simulink model "ECU_Arch0"  (R2022b)
settings: Solver=FixedStepDiscrete  StartTime=0.0  StopTime=10.0  RelTol=1e-3
model workspace (MAT data in the model file):
  AlignmentIdRef = Simulink.Parameter
  AlignmentIdRef.Value = 0.3
  AlignmentIdRef.Description = 'The required IdRef ( which applaies a voltage vector) to aligne the rotor to detect the encoder or resolver offset'
  AlignmentIdRef.DataType = 'single'
  AlignmentIdRef.Min = 0.1
  AlignmentIdRef.Max = 100
  AlignmentIdRef.DocUnits = 'A'
  AlignmentIdRef.Complexity = 'real'
  AlignmentIdRef.Dimensions = [1 1]
  Alignment_ReqTime_sec = Simulink.Parameter
  Alignment_ReqTime_sec.Value = 3
  Alignment_ReqTime_sec.DataType = 'single'
  Alignment_ReqTime_sec.Min = 0
  Alignment_ReqTime_sec.Max = 20
  Alignment_ReqTime_sec.Complexity = 'real'
  Alignment_ReqTime_sec.Dimensions = [1 1]
  AliveCounterStartGD = Simulink.Signal
  AliveCounterStartGD.Description = 'Alive counter to check the length of the Init of GateDriver'
  AliveCounterStartGD.DataType = 'single'
  AliveCounterStartGD.Min = -1000000
  AliveCounterStartGD.Max = 1000000
  AliveCounterStartGD.DocUnits = '-'
  AliveCounterStartGD.Dimensions = -1
  AliveCounterStartGD.DimensionsMode = 'auto'
  AliveCounterStartGD.Complexity = 'auto'
  AliveCounterStartGD.SampleTime = -1
  AliveCounterStartGD.SamplingMode = 'auto'
  AliveCounterStartGD.InitialValue = '0'
  AngleChangeDir = Simulink.Parameter
  AngleChangeDir.Value = 1
  AngleChangeDir.Description = 'It can be used to change the direction of the postion signal, but by default = 1'
  AngleChangeDir.DataType = 'single'
  AngleChangeDir.Min = -1
  AngleChangeDir.Max = 1
  AngleChangeDir.Complexity = 'real'
  AngleChangeDir.Dimensions = [1 1]
  C_LST = 0.0001
  CtrlMode = Simulink.Parameter
  CtrlMode.Value = 1
  CtrlMode.DataType = 'single'
  CtrlMode.Min = 0
  CtrlMode.Max = 1
  CtrlMode.Complexity = 'real'
  CtrlMode.Dimensions = [1 1]
  DelayTimeAfterOL_sec = Simulink.Parameter
  DelayTimeAfterOL_sec.Value = 5
  DelayTimeAfterOL_sec.DataType = 'single'
  DelayTimeAfterOL_sec.Min = 0
  DelayTimeAfterOL_sec.Max = 100
  DelayTimeAfterOL_sec.Complexity = 'real'
  DelayTimeAfterOL_sec.Dimensions = [1 1]
  DisablePWM = Simulink.Parameter
  DisablePWM.Value = 0
  DisablePWM.Description = 'Disable the PWM during the Rotor Offset Calibration'
  DisablePWM.DataType = 'single'
  DisablePWM.Min = 0
  DisablePWM.Max = 1
  DisablePWM.Complexity = 'real'
  DisablePWM.Dimensions = [1 1]
  DisablePWM_Selector = Simulink.Parameter
  DisablePWM_Selector.Value = 0
  DisablePWM_Selector.Description = 'select either without or with Disable the PWM during the Rotor Offset Calibration'
  DisablePWM_Selector.DataType = 'uint8'
  DisablePWM_Selector.Min = 0
  DisablePWM_Selector.Max = 1
  DisablePWM_Selector.DocUnits = '-'
  DisablePWM_Selector.Complexity = 'real'
  DisablePWM_Selector.Dimensions = [1 1]
  ExecutionTimeFastLoop_FOC = Simulink.Parameter
  ExecutionTimeFastLoop_FOC.Value = 0
  ExecutionTimeFastLoop_FOC.Description = 'to measure the execution time of the subsystem'
  ExecutionTimeFastLoop_FOC.DataType = 'single'
  ExecutionTimeFastLoop_FOC.Min = 0
  ExecutionTimeFastLoop_FOC.Max = 1000000
  ExecutionTimeFastLoop_FOC.Complexity = 'real'
  ExecutionTimeFastLoop_FOC.Dimensions = [1 1]
  IDcFilterConst = Simulink.Parameter
  IDcFilterConst.Value = 0.001
  IDcFilterConst.Description = 'Time constant of the FIR IDc current filter '
  IDcFilterConst.DataType = 'single'
  IDcFilterConst.Min = 0
  IDcFilterConst.Max = 1
  IDcFilterConst.Complexity = 'real'
  IDcFilterConst.Dimensions = [1 1]
  IDcFilterSelector = Simulink.Parameter
  IDcFilterSelector.Value = 0
  IDcFilterSelector.Description = 'Switch to select one of the applied IDc current filter '
  IDcFilterSelector.DataType = 'uint16'
  IDcFilterSelector.Min = 0
  IDcFilterSelector.Max = 1
  IDcFilterSelector.Complexity = 'real'
  IDcFilterSelector.Dimensions = [1 1]
  IDcOvercurrent = Simulink.Parameter
  IDcOvercurrent.Value = 5
  IDcOvercurrent.Description = 'value of the overcurrent'
  IDcOvercurrent.DataType = 'single'
  IDcOvercurrent.Min = 0.1
  IDcOvercurrent.Max = 100
  IDcOvercurrent.DocUnits = 'A'
  IDcOvercurrent.Complexity = 'real'
  IDcOvercurrent.Dimensions = [1 1]
  IDcOvercurrentAlignment = Simulink.Parameter
  IDcOvercurrentAlignment.Value = 6
  IDcOvercurrentAlignment.Description = 'Idc overcurrent limit during rotor alignment to detect the encoder or resolver offset'
  IDcOvercurrentAlignment.DataType = 'single'
  IDcOvercurrentAlignment.Min = 0.1
  IDcOvercurrentAlignment.Max = 100
  IDcOvercurrentAlignment.DocUnits = 'A'
  IDcOvercurrentAlignment.Complexity = 'real'
  IDcOvercurrentAlignment.Dimensions = [1 1]
  IQ_REF = Simulink.Signal
  IQ_REF.Description = 'The reference iq'
  IQ_REF.DataType = 'single'
  IQ_REF.Min = -100
  IQ_REF.Max = 100
  IQ_REF.DocUnits = 'A'
  IQ_REF.Dimensions = -1
  IQ_REF.DimensionsMode = 'auto'
  IQ_REF.Complexity = 'real'
  IQ_REF.SampleTime = -1
  IQ_REF.SamplingMode = 'auto'
  IQ_REF.InitialValue = '0'
  IQ_REF_MAX = Simulink.Parameter
  IQ_REF_MAX.Value = 2.3
  IQ_REF_MAX.Description = 'Maximum allowed Iq current to limit the output of the speed controller'
  IQ_REF_MAX.DataType = 'single'
  IQ_REF_MAX.Min = -100
  IQ_REF_MAX.Max = 100
  IQ_REF_MAX.DocUnits = 'A'
  IQ_REF_MAX.Complexity = 'real'
  IQ_REF_MAX.Dimensions = [1 1]
  I_MAX = Simulink.Parameter
  I_MAX.Value = 20.625
  I_MAX.Description = 'Maximum current used for current measurement scaling calibration'
  I_MAX.DataType = 'single'
  I_MAX.Min = -100
  I_MAX.Max = 100
  I_MAX.DocUnits = 'A'
  I_MAX.Complexity = 'real'
  I_MAX.Dimensions = [1 1]
  KiId = Simulink.Parameter
  KiId.Value = 0.5
  KiId.Description = 'proportional parameter Kp of the ID-current controller'
  KiId.DataType = 'single'
  KiId.Min = 0
  KiId.Max = 1000
  KiId.Complexity = 'real'
  KiId.Dimensions = [1 1]
  KiIq = Simulink.Parameter
  KiIq.Value = 0.5
  KiIq.Description = 'proportional parameter Kp of the IQ-current controller'
  KiIq.DataType = 'single'
  KiIq.Min = 0
  KiIq.Max = 1000
  KiIq.Complexity = 'real'
  KiIq.Dimensions = [1 1]
  KiSpd = Simulink.Parameter
  KiSpd.Value = 1
  KiSpd.Description = 'propotinal factor of speed controller'
  KiSpd.DataType = 'single'
  KiSpd.Min = 0
  KiSpd.Max = 1000
  KiSpd.Complexity = 'real'
  KiSpd.Dimensions = [1 1]
  KiSpdOrg = Simulink.Parameter
  KiSpdOrg.Value = 2.2316799098e-05
  KiSpdOrg.Description = 'propotinal factor of speed controller'
  KiSpdOrg.DataType = 'single'
  KiSpdOrg.Min = 0
  KiSpdOrg.Max = 1000
  KiSpdOrg.Complexity = 'real'
  KiSpdOrg.Dimensions = [1 1]
  KpId = Simulink.Parameter
  KpId.Value = 0.3
  KpId.Description = 'proportional parameter Kp of the ID-current controller'
  KpId.DataType = 'single'
  KpId.Min = 0
  KpId.Max = 1000
  KpId.Complexity = 'real'
  KpId.Dimensions = [1 1]
  KpIq = Simulink.Parameter
  KpIq.Value = 0.3
  KpIq.Description = 'proportional parameter Kp of the IQ-current controller'
  KpIq.DataType = 'single'
  KpIq.Min = 0
  KpIq.Max = 1000
  KpIq.Complexity = 'real'
  KpIq.Dimensions = [1 1]
  KpSpd = Simulink.Parameter
  KpSpd.Value = 1.5
  KpSpd.Description = 'propotinal factor of speed controller'
  KpSpd.DataType = 'single'
  KpSpd.Min = 0
  KpSpd.Max = 1000
  KpSpd.Complexity = 'real'
  KpSpd.Dimensions = [1 1]
  KpSpdOrg = Simulink.Parameter
  KpSpdOrg.Value = 0.0142073155617
  KpSpdOrg.Description = 'propotinal factor of speed controller'
  KpSpdOrg.DataType = 'single'
  KpSpdOrg.Min = 0
  KpSpdOrg.Max = 1000
  KpSpdOrg.Complexity = 'real'
  KpSpdOrg.Dimensions = [1 1]
  Low_TQLimit_SpdCtrl = Simulink.Parameter
  Low_TQLimit_SpdCtrl.Value = -0.12
  Low_TQLimit_SpdCtrl.DataType = 'single'
  Low_TQLimit_SpdCtrl.Min = -10
  Low_TQLimit_SpdCtrl.Max = 0
  Low_TQLimit_SpdCtrl.Complexity = 'real'
  Low_TQLimit_SpdCtrl.Dimensions = [1 1]
  Low_TQLimit_TqCtrl = Simulink.Parameter
  Low_TQLimit_TqCtrl.Value = -0.04
  Low_TQLimit_TqCtrl.DataType = 'single'
  Low_TQLimit_TqCtrl.Min = -10
  Low_TQLimit_TqCtrl.Max = 0
  Low_TQLimit_TqCtrl.Complexity = 'real'
  Low_TQLimit_TqCtrl.Dimensions = [1 1]
  MaxSpdLimit = Simulink.Parameter
  MaxSpdLimit.Value = 199
  MaxSpdLimit.Description = 'Maximum Allowed Speed'
  MaxSpdLimit.DataType = 'single'
  MaxSpdLimit.Min = -524
  MaxSpdLimit.Max = 524
  MaxSpdLimit.DocUnits = 'rad/sec'
  MaxSpdLimit.Complexity = 'real'
  MaxSpdLimit.Dimensions = [1 1]
  Nmax = Simulink.Parameter
  Nmax.Value = 6000
  Nmax.Description = 'polpair'
  Nmax.DataType = 'int32'
  Nmax.Min = 1
  Nmax.Max = 20000
  Nmax.DocUnits = '-'
  Nmax.Complexity = 'real'
  Nmax.Dimensions = [1 1]
  OL_IDcOvercurrent = Simulink.Parameter
  OL_IDcOvercurrent.Value = 5.5
  OL_IDcOvercurrent.DataType = 'single'
  OL_IDcOvercurrent.Min = 0
  OL_IDcOvercurrent.Max = 7
  OL_IDcOvercurrent.Complexity = 'real'
  OL_IDcOvercurrent.Dimensions = [1 1]
  OL_ReqTime_sec = Simulink.Parameter
  OL_ReqTime_sec.Value = 1
  OL_ReqTime_sec.DataType = 'single'
  OL_ReqTime_sec.Min = 0
  OL_ReqTime_sec.Max = 20
  OL_ReqTime_sec.Complexity = 'real'
  OL_ReqTime_sec.Dimensions = [1 1]
  OffsetSelector = Simulink.Parameter
  OffsetSelector.Value = 0
  OffsetSelector.Description = 'switch to select the finial rotor offset either add to the actual rotor position or substract from the actual rotor position'
  OffsetSelector.DataType = 'uint8'
  OffsetSelector.Min = 0
  OffsetSelector.Max = 1
  OffsetSelector.Complexity = 'real'
  OffsetSelector.Dimensions = [1 1]
  PISpdControllerSelector = Simulink.Parameter
  PISpdControllerSelector.Value = 0
  PISpdControllerSelector.Description = 'selector to test the correct PI speed controller'
  PISpdControllerSelector.DataType = 'uint8'
  PISpdControllerSelector.Min = 0
  PISpdControllerSelector.Max = 1
  PISpdControllerSelector.Complexity = 'real'
  PISpdControllerSelector.Dimensions = [1 1]
  PMflux = Simulink.Parameter
  PMflux.Value = 0.0064
  PMflux.DataType = 'single'
  PMflux.Min = 0
  PMflux.Max = 10
  PMflux.Complexity = 'real'
  PMflux.Dimensions = [1 1]
  PP = Simulink.Parameter
  PP.Value = 4
  PP.Description = 'polpair'
  PP.DataType = 'int32'
  PP.Min = 1
  PP.Max = 10
  PP.DocUnits = '-'
  PP.Complexity = 'real'
  PP.Dimensions = [1 1]
  PWMDutyCycle_A = Simulink.Signal
  PWMDutyCycle_A.Description = 'Input of the PWM Phase A '
  PWMDutyCycle_A.DataType = 'single'
  PWMDutyCycle_A.Min = -100
  PWMDutyCycle_A.Max = 100
  PWMDutyCycle_A.DocUnits = '-'
  PWMDutyCycle_A.Dimensions = -1
  PWMDutyCycle_A.DimensionsMode = 'auto'
  PWMDutyCycle_A.Complexity = 'real'
  PWMDutyCycle_A.SampleTime = -1
  PWMDutyCycle_A.SamplingMode = 'auto'
  PWMDutyCycle_A.InitialValue = '0'
  PWMDutyCycle_B = Simulink.Signal
  PWMDutyCycle_B.Description = 'Input of the PWM Phase B '
  PWMDutyCycle_B.DataType = 'single'
  PWMDutyCycle_B.Min = -100
  PWMDutyCycle_B.Max = 100
  PWMDutyCycle_B.DocUnits = '-'
  PWMDutyCycle_B.Dimensions = -1
  PWMDutyCycle_B.DimensionsMode = 'auto'
  PWMDutyCycle_B.Complexity = 'real'
  PWMDutyCycle_B.SampleTime = -1
  PWMDutyCycle_B.SamplingMode = 'auto'
  PWMDutyCycle_B.InitialValue = '0'
  PWMDutyCycle_C = Simulink.Signal
  PWMDutyCycle_C.Description = 'Input of the PWM Phase C '
  PWMDutyCycle_C.DataType = 'single'
  PWMDutyCycle_C.Min = -100
  PWMDutyCycle_C.Max = 100
  PWMDutyCycle_C.DocUnits = '-'
  PWMDutyCycle_C.Dimensions = -1
  PWMDutyCycle_C.DimensionsMode = 'auto'
  PWMDutyCycle_C.Complexity = 'real'
  PWMDutyCycle_C.SampleTime = -1
  PWMDutyCycle_C.SamplingMode = 'auto'
  PWMDutyCycle_C.InitialValue = '0'
  PhA_Offset = Simulink.Parameter
  PhA_Offset.Value = 20.625
  PhA_Offset.Description = 'Offset current value of phase A, which used for current calibration'
  PhA_Offset.DataType = 'single'
  PhA_Offset.Min = -100
  PhA_Offset.Max = 100
  PhA_Offset.DocUnits = 'A'
  PhA_Offset.Complexity = 'real'
  PhA_Offset.Dimensions = [1 1]
  PhB_Offset = Simulink.Parameter
  PhB_Offset.Value = 20.625
  PhB_Offset.Description = 'Offset current value of phase B, which used for current calibration'
  PhB_Offset.DataType = 'single'
  PhB_Offset.Min = -100
  PhB_Offset.Max = 100
  PhB_Offset.DocUnits = 'A'
  PhB_Offset.Complexity = 'real'
  PhB_Offset.Dimensions = [1 1]
  RotorOffsetMotor1_Selector = Simulink.Parameter
  RotorOffsetMotor1_Selector.Value = 1
  RotorOffsetMotor1_Selector.Description = 'Feedback when the rotor offset of motor1 is completed '
  RotorOffsetMotor1_Selector.DataType = 'single'
  RotorOffsetMotor1_Selector.Min = 0
  RotorOffsetMotor1_Selector.Max = 1
  RotorOffsetMotor1_Selector.DocUnits = '-'
  RotorOffsetMotor1_Selector.Complexity = 'real'
  RotorOffsetMotor1_Selector.Dimensions = [1 1]
  RotorOffsetMotor2_Selector = Simulink.Parameter
  RotorOffsetMotor2_Selector.Value = 1
  RotorOffsetMotor2_Selector.Description = 'Feedback when the rotor offset of motor2 is completed '
  RotorOffsetMotor2_Selector.DataType = 'single'
  RotorOffsetMotor2_Selector.Min = 0
  RotorOffsetMotor2_Selector.Max = 1
  RotorOffsetMotor2_Selector.DocUnits = '-'
  RotorOffsetMotor2_Selector.Complexity = 'real'
  RotorOffsetMotor2_Selector.Dimensions = [1 1]
  SPEED_CMD = Simulink.Parameter
  SPEED_CMD.Value = 500
  SPEED_CMD.Description = 'Reference speed in rpm'
  SPEED_CMD.DataType = 'single'
  SPEED_CMD.Min = -2200
  SPEED_CMD.Max = 2200
  SPEED_CMD.Complexity = 'real'
  SPEED_CMD.Dimensions = [1 1]
  SPEED_DOWN_INC = Simulink.Parameter
  SPEED_DOWN_INC.Value = 50
  SPEED_DOWN_INC.Description = 'Gain used to decrease the reference speed (SPEED_CMD)using push botton on the MPC5744P board '
  SPEED_DOWN_INC.DataType = 'single'
  SPEED_DOWN_INC.Min = -1000
  SPEED_DOWN_INC.Max = 1000
  SPEED_DOWN_INC.Complexity = 'real'
  SPEED_DOWN_INC.Dimensions = [1 1]
  SPEED_LOOP_CNTR = Simulink.Parameter
  SPEED_LOOP_CNTR.Value = 10
  SPEED_LOOP_CNTR.Description = 'speed loop counter, which used to determine who many current loops are over to recall the speed loop  '
  SPEED_LOOP_CNTR.DataType = 'single'
  SPEED_LOOP_CNTR.Min = -1000
  SPEED_LOOP_CNTR.Max = 1000
  SPEED_LOOP_CNTR.Complexity = 'real'
  SPEED_LOOP_CNTR.Dimensions = [1 1]
  SPEED_UP_INC = Simulink.Parameter
  SPEED_UP_INC.Value = 50
  SPEED_UP_INC.Description = 'Gain used to decrease the reference speed (SPEED_CMD)using push botton on the MPC5744P board '
  SPEED_UP_INC.DataType = 'single'
  SPEED_UP_INC.Min = -1000
  SPEED_UP_INC.Max = 1000
  SPEED_UP_INC.Complexity = 'real'
  SPEED_UP_INC.Dimensions = [1 1]
  S_LST = 0.001
  Sig = Simulink.Signal
  Sig.DataType = 'auto'
  Sig.Dimensions = -1
  Sig.DimensionsMode = 'auto'
  Sig.Complexity = 'auto'
  Sig.SampleTime = -1
  Sig.SamplingMode = 'auto'
  SpdChangeDir = Simulink.Parameter
  SpdChangeDir.Value = 1
  SpdChangeDir.Description = 'It can be used to change the direction of the speed signal, but by default = 1'
  SpdChangeDir.DataType = 'single'
  SpdChangeDir.Min = -1
  SpdChangeDir.Max = 1
  SpdChangeDir.Complexity = 'real'
  SpdChangeDir.Dimensions = [1 1]
  SpdDecreasingStep = Simulink.Parameter
  SpdDecreasingStep.Value = 0.01
  SpdDecreasingStep.DataType = 'single'
  SpdDecreasingStep.Min = 0
  SpdDecreasingStep.Max = 100
  SpdDecreasingStep.Complexity = 'real'
  SpdDecreasingStep.Dimensions = [1 1]
  SpdFilterConst = Simulink.Parameter
  SpdFilterConst.Value = 0.0005
  SpdFilterConst.Description = 'Time constant of the FIR speed filter '
  SpdFilterConst.DataType = 'single'
  SpdFilterConst.Min = 0
  SpdFilterConst.Max = 1
  SpdFilterConst.Complexity = 'real'
  SpdFilterConst.Dimensions = [1 1]
  SpeedAct = Simulink.Signal
  SpeedAct.Description = 'The measured actual speed in rad/sec'
  SpeedAct.DataType = 'single'
  SpeedAct.Min = -200000
  SpeedAct.Max = 20000
  SpeedAct.DocUnits = 'rad/sec'
  SpeedAct.Dimensions = -1
  SpeedAct.DimensionsMode = 'auto'
  SpeedAct.Complexity = 'real'
  SpeedAct.SampleTime = -1
  SpeedAct.SamplingMode = 'auto'
  SpeedAct.InitialValue = '0'
  SpeedActRpm = Simulink.Signal
  SpeedActRpm.Description = 'The measured actual speed in rpm'
  SpeedActRpm.DataType = 'single'
  SpeedActRpm.Min = -20000
  SpeedActRpm.Max = 20000
  SpeedActRpm.DocUnits = 'rpm'
  SpeedActRpm.Dimensions = -1
  SpeedActRpm.DimensionsMode = 'auto'
  SpeedActRpm.Complexity = 'real'
  SpeedActRpm.SampleTime = -1
  SpeedActRpm.SamplingMode = 'auto'
  SpeedActRpm.InitialValue = '0'
  SpeedCmd = Simulink.Signal
  SpeedCmd.Description = 'The speed command in rpm'
  SpeedCmd.DataType = 'single'
  SpeedCmd.Min = -20000
  SpeedCmd.Max = 20000
  SpeedCmd.DocUnits = 'rad/sec'
  SpeedCmd.Dimensions = -1
  SpeedCmd.DimensionsMode = 'auto'
  SpeedCmd.Complexity = 'real'
  SpeedCmd.SampleTime = -1
  SpeedCmd.SamplingMode = 'auto'
  SpeedCmd.InitialValue = '0'
  SpeedRef = Simulink.Signal
  SpeedRef.Description = 'The reference speed in rad/sec after filtered SPEED_Cmd'
  SpeedRef.DataType = 'single'
  SpeedRef.Min = -2000
  SpeedRef.Max = 2000
  SpeedRef.DocUnits = 'rad/sec'
  SpeedRef.Dimensions = -1
  SpeedRef.DimensionsMode = 'auto'
  SpeedRef.Complexity = 'real'
  SpeedRef.SampleTime = -1
  SpeedRef.SamplingMode = 'auto'
  SpeedRef.InitialValue = '0'
  SpeedThresholdOvercurrent = Simulink.Parameter
  SpeedThresholdOvercurrent.Value = 0
  SpeedThresholdOvercurrent.Description = 'This is speed threshold in rad/sec, which is used to switch the another IDc overcurrent value to meet the high current of Teknic M-2310P-LN-04K during the rotor alignment'
  SpeedThresholdOvercurrent.DataType = 'single'
  SpeedThresholdOvercurrent.Min = 0
  SpeedThresholdOvercurrent.Max = 40
  SpeedThresholdOvercurrent.Complexity = 'real'
  SpeedThresholdOvercurrent.Dimensions = [1 1]
  ThetaOffsetIncEncoder = Simulink.Signal
  ThetaOffsetIncEncoder.Description = 'The detected rotor offset of the incremental encoder'
  ThetaOffsetIncEncoder.DataType = 'single'
  ThetaOffsetIncEncoder.Min = -1000
  ThetaOffsetIncEncoder.Max = 1000
  ThetaOffsetIncEncoder.DocUnits = 'rad'
  ThetaOffsetIncEncoder.Dimensions = -1
  ThetaOffsetIncEncoder.DimensionsMode = 'auto'
  ThetaOffsetIncEncoder.Complexity = 'real'
  ThetaOffsetIncEncoder.SampleTime = -1
  ThetaOffsetIncEncoder.SamplingMode = 'auto'
  ThetaOffsetIncEncoder.InitialValue = '0'
  Torque_Ref = Simulink.Signal
  Torque_Ref.Description = 'The reference torque'
  Torque_Ref.DataType = 'single'
  Torque_Ref.Min = -100
  Torque_Ref.Max = 100
  Torque_Ref.DocUnits = 'Nm'
  Torque_Ref.Dimensions = -1
  Torque_Ref.DimensionsMode = 'auto'
  Torque_Ref.Complexity = 'auto'
  Torque_Ref.SampleTime = -1
  Torque_Ref.SamplingMode = 'auto'
  Torque_Ref.InitialValue = '0'
  TqCtrlRef = Simulink.Parameter
  TqCtrlRef.Value = 0.03
  TqCtrlRef.Description = 'Reference Torque'
  TqCtrlRef.DataType = 'single'
  TqCtrlRef.Min = -3
  TqCtrlRef.Max = 3
  TqCtrlRef.DocUnits = 'Nm'
  TqCtrlRef.Complexity = 'real'
  TqCtrlRef.Dimensions = [1 1]
  TqCtrlSwitch = Simulink.Parameter
  TqCtrlSwitch.Value = 0
  TqCtrlSwitch.Description = 'Switch to select Speed Control "0" or Torque Control "1"'
  TqCtrlSwitch.DataType = 'boolean'
  TqCtrlSwitch.Min = 0
  TqCtrlSwitch.Max = 1
  TqCtrlSwitch.Complexity = 'real'
  TqCtrlSwitch.Dimensions = [1 1]
  TqDecreasingStep = Simulink.Parameter
  TqDecreasingStep.Value = 3e-06
  TqDecreasingStep.DataType = 'single'
  TqDecreasingStep.Min = 0
  TqDecreasingStep.Max = 100
  TqDecreasingStep.Complexity = 'real'
  TqDecreasingStep.Dimensions = [1 1]
  TqFilterConst = Simulink.Parameter
  TqFilterConst.Value = 0.001
  TqFilterConst.Description = 'Time constant of the FIR torque filter '
  TqFilterConst.DataType = 'single'
  TqFilterConst.Min = 0
  TqFilterConst.Max = 1
  TqFilterConst.DocUnits = '-'
  TqFilterConst.Complexity = 'real'
  TqFilterConst.Dimensions = [1 1]
  TrgTime = Simulink.Parameter
  TrgTime.Value = 10000
  TrgTime.DataType = 'single'
  TrgTime.Min = 0
  TrgTime.Max = 10000000
  TrgTime.Complexity = 'real'
  TrgTime.Dimensions = [1 1]
  UAlpha = Simulink.Signal
  UAlpha.Description = 'voltage on alpha axis related to the Alpha-Beta coordination system'
  UAlpha.DataType = 'single'
  UAlpha.Min = -500
  UAlpha.Max = 500
  UAlpha.DocUnits = 'V'
  UAlpha.Dimensions = -1
  UAlpha.DimensionsMode = 'auto'
  UAlpha.Complexity = 'real'
  UAlpha.SampleTime = -1
  UAlpha.SamplingMode = 'auto'
  UAlpha.InitialValue = '0'
  UBeta = Simulink.Signal
  UBeta.Description = 'voltage on beta axis related to the Alpha-Beta coordination system'
  UBeta.DataType = 'single'
  UBeta.Min = -500
  UBeta.Max = 500
  UBeta.DocUnits = 'V'
  UBeta.Dimensions = -1
  UBeta.DimensionsMode = 'auto'
  UBeta.Complexity = 'real'
  UBeta.SampleTime = -1
  UBeta.SamplingMode = 'auto'
  UBeta.InitialValue = '0'
  UP_TQLimit_SpdCtrl = Simulink.Parameter
  UP_TQLimit_SpdCtrl.Value = 0.12
  UP_TQLimit_SpdCtrl.DataType = 'single'
  UP_TQLimit_SpdCtrl.Min = 0
  UP_TQLimit_SpdCtrl.Max = 10
  UP_TQLimit_SpdCtrl.Complexity = 'real'
  UP_TQLimit_SpdCtrl.Dimensions = [1 1]
  UP_TQLimit_TqCtrl = Simulink.Parameter
  UP_TQLimit_TqCtrl.Value = 0.04
  UP_TQLimit_TqCtrl.DataType = 'single'
  UP_TQLimit_TqCtrl.Min = 0
  UP_TQLimit_TqCtrl.Max = 10
  UP_TQLimit_TqCtrl.Complexity = 'real'
  UP_TQLimit_TqCtrl.Dimensions = [1 1]
  VDC_OVERVOLTAGE = Simulink.Parameter
  VDC_OVERVOLTAGE.Value = 18
  VDC_OVERVOLTAGE.Description = 'Overvoltage protection  '
  VDC_OVERVOLTAGE.DataType = 'single'
  VDC_OVERVOLTAGE.Min = -1000
  VDC_OVERVOLTAGE.Max = 1000
  VDC_OVERVOLTAGE.Complexity = 'real'
  VDC_OVERVOLTAGE.Dimensions = [1 1]
  VDC_UNDERVOLTAGE = Simulink.Parameter
  VDC_UNDERVOLTAGE.Value = 8
  VDC_UNDERVOLTAGE.Description = 'Undervoltage protection '
  VDC_UNDERVOLTAGE.DataType = 'single'
  VDC_UNDERVOLTAGE.Min = -1000
  VDC_UNDERVOLTAGE.Max = 1000
  VDC_UNDERVOLTAGE.Complexity = 'real'
  VDC_UNDERVOLTAGE.Dimensions = [1 1]
  WaitingTimeAfterAlignment_sec = Simulink.Parameter
  WaitingTimeAfterAlignment_sec.Value = 5
  WaitingTimeAfterAlignment_sec.DataType = 'single'
  WaitingTimeAfterAlignment_sec.Min = 0
  WaitingTimeAfterAlignment_sec.Max = 100
  WaitingTimeAfterAlignment_sec.Complexity = 'real'
  WaitingTimeAfterAlignment_sec.Dimensions = [1 1]
undefined symbols (not defined in the file): D1, P
settings Model: Creator=MAAM  LastModifiedBy=MAAM
settings OptimizationCC: DefaultParameterBehavior=Inlined  EnhancedBackFolding=on  PassReuseOutputArgsAs=Individual arguments  ZeroExternalMemoryAtStartup=off  ZeroInternalMemoryAtStartup=off  OptimizeBlockOrder=speed  DifferentSizesBufferReuse=on  OptimizationCustomize=off  EfficientTunableParamExpr=on
settings DebuggingCC: ParameterTunabilityLossMsg=error
settings SFSimCC: MATLABDynamicMemAlloc=off
settings RTWCC: Description=Model Based Design Toolbox MPC57xx Code Generation Target  SystemTargetFile=mbd_mpc574x.tlc  MakeCommand=mbd_mpc574x_make_rtw COPY_MDLREF_INCLUDES=0  TemplateMakefile=mbd_mpc574x.tmf
settings CodeAppCC: ForceParamTrailComments=on  IgnoreCustomStorageClasses=off  OperatorAnnotations=on  SimulinkDataObjDesc=on  SFDataObjDesc=on  InsertBlockDesc=on
settings STFCustomTargetCC: TargetLangStandard=C99 (ISO)  MultiwordLength=256  CombineOutputUpdateFcns=on  ERTCustomFileBanners=on  SupportContinuousTime=off  SupportNonInlinedSFcns=off  RemoveResetFunc=on  MATLABClassNameForMDSCustomization=Simulink.SoftwareTarget.ERTCustomization  SystemTargetFile=mbd_mpc574x.tlc
settings ERTTargetCC: TargetLangStandard=C99 (ISO)  ParMdlRefBuildCompliant=off  CompOptLevelCompliant=off  ConcurrentExecutionCompliant=off  ModelStepFunctionPrototypeControlCompliant=off  CPPClassGenCompliant=off  UseToolchainInfoCompliant=off  InlinedParameterPlacement=NonHierarchical  ERTCustomFileTemplate=example_file_process.tlc

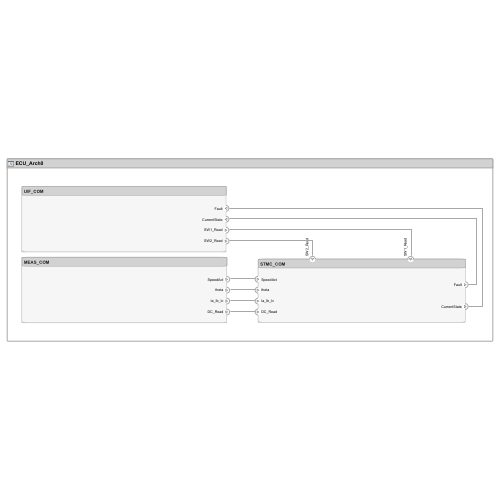
[thumbnail: Simulink's stored preview of the top-level diagram]
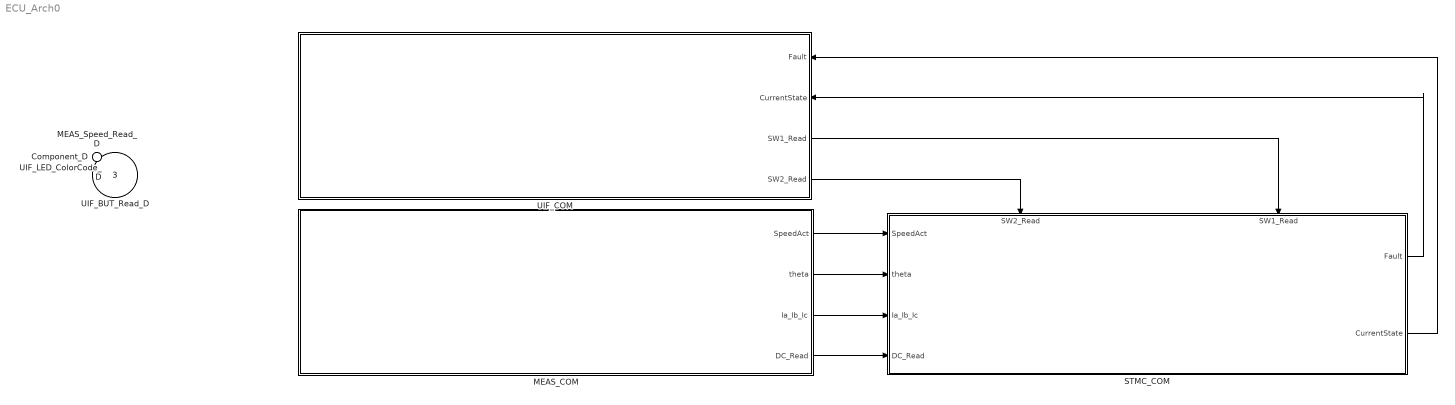
== system ECU_Arch0 ==
  MEAS_Speed_Read_D : Inport  OutputFunctionCall=on
  Component_D : Inport  Port=2  OutputFunctionCall=on
  UIF_BUT_Read_D : Inport  Port=3  OutputFunctionCall=on
  UIF_LED_ColorCode_D : Inport  Port=4  OutputFunctionCall=on
  MEAS_COM : Subsystem
      settings: PortSchema="{\"entries\":[{\"content\":{\"headerSize\":26,\"margin\":15,\"minimumSpacing\":25,\"sides\":[{\"content\":{\"connectorIds\":[]},\"type\":\"ConnectorPlacement.EquallySpacedRectSide\",\"uuid\":\"9fafbac4-d9ff-4bef-9686-25ce946f922a\"},{\"content\":{\"connectorIds\":[\"Out1\",\"Out2\",\"Out3\",\"Out4\"],\"side\":\"RIGHT\"},\"type\":\"ConnectorPlacement.EquallySpacedRectSide\",\"uuid\":\"64958763-52cc-4c3d-9da1-de7e7fca94ff\"},{\"content\":{\"connectorIds\":[],\"side\":\"TOP\"},\"type\":\"ConnectorPlacement.EquallySpacedRectSide\",\"uuid\":\"29c78429-a934-4b6b-906c-5a3963e1854a\"},{\"content\":{\"connectorIds\":[],\"side\":\"BOTTOM\"},\"type\":\"ConnectorPlacement.EquallySpacedRectSide\",\"uuid\":\"f9f9d59b-2161-4ff7-aea9-ea3466aa3e9c\"}]},\"type\":\"ConnectorPlacement.EquallySpacedConnector\",\"uuid\":\"b6b0d473-12c9-4a38-8dee-bffc8352e44f\"}],\"packageUris\":[\"http://schema.mathworks.com/mf0/Connector/R2020b\"],\"version\":\"1.0\"}"
  STMC_COM : Subsystem
      settings: PortSchema="{\"entries\":[{\"content\":{\"headerSize\":26,\"margin\":15,\"minimumSpacing\":25,\"sides\":[{\"content\":{\"connectorIds\":[\"In3\",\"In5\",\"In6\",\"In4\"]},\"type\":\"ConnectorPlacement.EquallySpacedRectSide\",\"uuid\":\"9fafbac4-d9ff-4bef-9686-25ce946f922a\"},{\"content\":{\"connectorIds\":[\"Out2\",\"Out1\"],\"side\":\"RIGHT\"},\"type\":\"ConnectorPlacement.EquallySpacedRectSide\",\"uuid\":\"64958763-52cc-4c3d-9da1-de7e7fca94ff\"},{\"content\":{\"connectorIds\":[\"In1\",\"In2\"],\"side\":\"TOP\"},\"type\":\"ConnectorPlacement.EquallySpacedRectSide\",\"uuid\":\"29c78429-a934-4b6b-906c-5a3963e1854a\"},{\"content\":{\"connectorIds\":[],\"side\":\"BOTTOM\"},\"type\":\"ConnectorPlacement.EquallySpacedRectSide\",\"uuid\":\"f9f9d59b-2161-4ff7-aea9-ea3466aa3e9c\"}]},\"type\":\"ConnectorPlacement.EquallySpacedConnector\",\"uuid\":\"b6b0d473-12c9-4a38-8dee-bffc8352e44f\"}],\"packageUris\":[\"http://schema.mathworks.com/mf0/Connector/R2020b\"],\"version\":\"1.0\"}"
  UIF_COM : Subsystem
      settings: PortSchema="{\"entries\":[{\"content\":{\"headerSize\":26,\"margin\":15,\"minimumSpacing\":25,\"sides\":[{\"content\":{\"connectorIds\":[]},\"type\":\"ConnectorPlacement.EquallySpacedRectSide\",\"uuid\":\"9fafbac4-d9ff-4bef-9686-25ce946f922a\"},{\"content\":{\"connectorIds\":[\"In2\",\"In1\",\"Out1\",\"Out2\"],\"side\":\"RIGHT\"},\"type\":\"ConnectorPlacement.EquallySpacedRectSide\",\"uuid\":\"64958763-52cc-4c3d-9da1-de7e7fca94ff\"},{\"content\":{\"connectorIds\":[],\"side\":\"TOP\"},\"type\":\"ConnectorPlacement.EquallySpacedRectSide\",\"uuid\":\"29c78429-a934-4b6b-906c-5a3963e1854a\"},{\"content\":{\"connectorIds\":[],\"side\":\"BOTTOM\"},\"type\":\"ConnectorPlacement.EquallySpacedRectSide\",\"uuid\":\"f9f9d59b-2161-4ff7-aea9-ea3466aa3e9c\"}]},\"type\":\"ConnectorPlacement.EquallySpacedConnector\",\"uuid\":\"b6b0d473-12c9-4a38-8dee-bffc8352e44f\"}],\"packageUris\":[\"http://schema.mathworks.com/mf0/Connector/R2020b\"],\"version\":\"1.0\"}"
  wires:
  MEAS_COM/1(SpeedAct) -> STMC_COM/3(SpeedAct)
  MEAS_COM/2(theta) -> STMC_COM/5(theta)
  MEAS_COM/3(Ia_Ib_Ic) -> STMC_COM/6(Ia_Ib_Ic)
  STMC_COM/1(CurrentState) -> UIF_COM/2(Fault)
  STMC_COM/2(Fault) -> UIF_COM/1(CurrentState)
  UIF_COM/2(SW2_Read) -> STMC_COM/1(SW2_Read)
  UIF_COM/1(SW1_Read) -> STMC_COM/2(SW1_Read)
  MEAS_COM/4(DC_Read) -> STMC_COM/4(DC_Read)

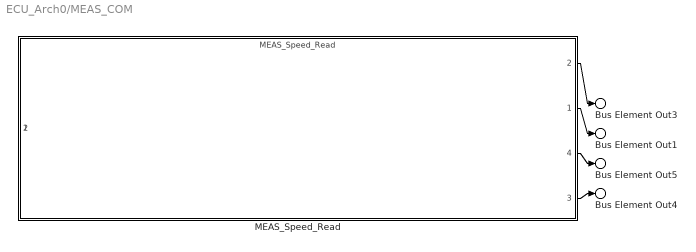
== system ECU_Arch0/MEAS_COM ==
  MEAS_Speed_Read : ModelReference  ModelNameDialog=MEAS_Speed_Read.slx  SimulationMode=Normal  ScheduleRates=on  ModelEventPortInfo=P:D1[-2][0][0]  ModelReferenceVersion=1.11
      settings: PortSchema="{\"entries\":[{\"content\":{\"headerSize\":38,\"margin\":15,\"minimumSpacing\":25,\"sides\":[{\"content\":{\"connectorIds\":[\"In1\"]},\"type\":\"ConnectorPlacement.EquallySpacedRectSide\",\"uuid\":\"9058249d-e940-4d4a-a6f5-813527d9e085\"},{\"content\":{\"connectorIds\":[\"Out2\",\"Out1\",\"Out4\",\"Out3\"],\"side\":\"RIGHT\"},\"type\":\"ConnectorPlacement.EquallySpacedRectSide\",\"uuid\":\"a8e78085-bda8-476a-9df8-aa18e7304955\"},{\"content\":{\"connectorIds\":[],\"side\":\"TOP\"},\"type\":\"ConnectorPlacement.EquallySpacedRectSide\",\"uuid\":\"80c09573-2c5c-4731-8526-0cc3e38135f7\"},{\"content\":{\"connectorIds\":[\"In2\"],\"side\":\"HIDDEN\"},\"type\":\"ConnectorPlacement.EquallySpacedRectSide\",\"uuid\":\"c5d5123f-b5f0-4021-bf98-bc28477bc88a\"}]},\"type\":\"ConnectorPlacement.EquallySpacedConnector\",\"uuid\":\"1baa5a0e-f319-46de-91b9-61d8c186ad39\"}],\"packageUris\":[\"http://schema.mathworks.com/mf0/Connector/R2020b\"],\"version\":\"1.0\"}"
  Bus Element Out1 : Outport  PortName=SpeedAct
  Bus Element Out4 : Outport  Port=2  PortName=theta
  Bus Element Out3 : Outport  Port=3  PortName=Ia_Ib_Ic
  Bus Element Out5 : Outport  Port=4  PortName=DC_Read
  wires:
  MEAS_Speed_Read/1 -> Bus Element Out1/1
  MEAS_Speed_Read/3 -> Bus Element Out4/1
  MEAS_Speed_Read/4 -> Bus Element Out5/1
  MEAS_Speed_Read/2 -> Bus Element Out3/1

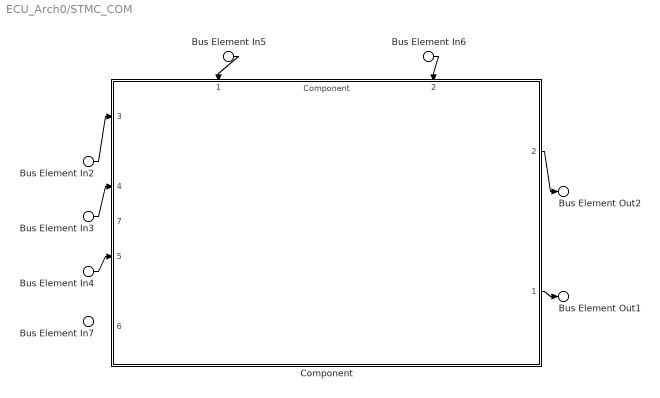
== system ECU_Arch0/STMC_COM ==
  Bus Element In5 : Inport  PortName=SW2_Read
  Bus Element In6 : Inport  Port=2  PortName=SW1_Read
  Bus Element In2 : Inport  Port=3  PortName=SpeedAct
  Bus Element In7 : Inport  Port=4  PortName=DC_Read
  Bus Element In3 : Inport  Port=5  PortName=theta
  Bus Element In4 : Inport  Port=6  PortName=Ia_Ib_Ic
  Component : ModelReference  ModelNameDialog=Component.slx  SimulationMode=Normal  ScheduleRates=on  ModelEventPortInfo=P:D1[-2][0][0]  ModelReferenceVersion=1.7
      settings: PortSchema="{\"entries\":[{\"content\":{\"headerSize\":38,\"margin\":15,\"minimumSpacing\":25,\"sides\":[{\"content\":{\"connectorIds\":[\"In3\",\"In4\",\"In5\",\"In6\"]},\"type\":\"ConnectorPlacement.EquallySpacedRectSide\",\"uuid\":\"9058249d-e940-4d4a-a6f5-813527d9e085\"},{\"content\":{\"connectorIds\":[\"Out2\",\"Out1\"],\"side\":\"RIGHT\"},\"type\":\"ConnectorPlacement.EquallySpacedRectSide\",\"uuid\":\"a8e78085-bda8-476a-9df8-aa18e7304955\"},{\"content\":{\"connectorIds\":[\"In1\",\"In2\"],\"side\":\"TOP\"},\"type\":\"ConnectorPlacement.EquallySpacedRectSide\",\"uuid\":\"80c09573-2c5c-4731-8526-0cc3e38135f7\"},{\"content\":{\"connectorIds\":[],\"side\":\"BOTTOM\"},\"type\":\"ConnectorPlacement.EquallySpacedRectSide\",\"uuid\":\"044f03b7-32e1-4176-8973-56ac0a1beaf0\"},{\"content\":{\"connectorIds\":[\"In7\"],\"side\":\"HIDDEN\"},\"type\":\"ConnectorPlacement.EquallySpacedRectSide\",\"uuid\":\"2588ea74-19e8-4cfe-b4e7-85ca69cec0cb\"}]},\"type\":\"ConnectorPlacement.EquallySpacedConnector\",\"uuid\":\"1baa5a0e-f319-46de-91b9-61d8c186ad39\"}],\"packageUris\":[\"http://schema.mathworks.com/mf0/Connector/R2020b\"],\"version\":\"1.0\"}"
  Bus Element Out1 : Outport  PortName=CurrentState
  Bus Element Out2 : Outport  Port=2  PortName=Fault
  wires:
  Bus Element In6/1 -> Component/2
  Bus Element In5/1 -> Component/1
  Component/1 -> Bus Element Out1/1
  Component/2 -> Bus Element Out2/1
  Bus Element In3/1 -> Component/4
  Bus Element In2/1 -> Component/3
  Bus Element In4/1 -> Component/5

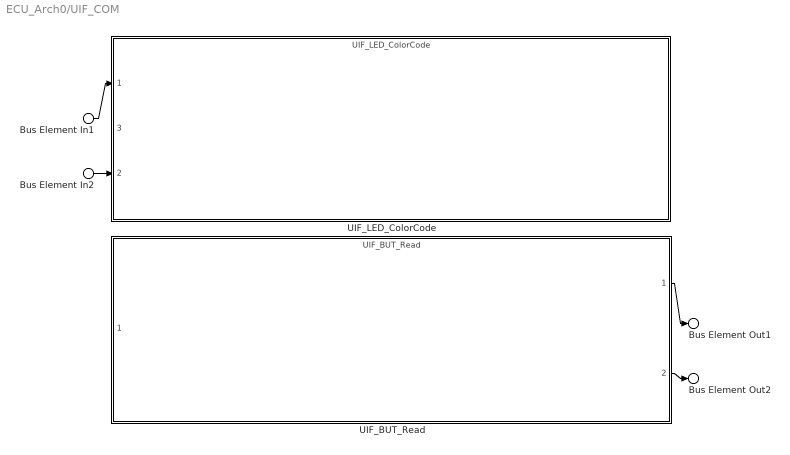
== system ECU_Arch0/UIF_COM ==
  Bus Element In1 : Inport  PortName=CurrentState
  Bus Element In2 : Inport  Port=2  PortName=Fault
  UIF_BUT_Read : ModelReference  ModelNameDialog=UIF_BUT_Read  SimulationMode=Normal  ScheduleRates=on  ModelEventPortInfo=P:D1[-2][0][0]  ModelReferenceVersion=1.4
      settings: PortSchema="{\"entries\":[{\"content\":{\"headerSize\":38,\"margin\":15,\"minimumSpacing\":25,\"sides\":[{\"content\":{\"connectorIds\":[]},\"type\":\"ConnectorPlacement.EquallySpacedRectSide\",\"uuid\":\"9fafbac4-d9ff-4bef-9686-25ce946f922a\"},{\"content\":{\"connectorIds\":[\"Out1\",\"Out2\"],\"side\":\"RIGHT\"},\"type\":\"ConnectorPlacement.EquallySpacedRectSide\",\"uuid\":\"64958763-52cc-4c3d-9da1-de7e7fca94ff\"},{\"content\":{\"connectorIds\":[],\"side\":\"TOP\"},\"type\":\"ConnectorPlacement.EquallySpacedRectSide\",\"uuid\":\"29c78429-a934-4b6b-906c-5a3963e1854a\"},{\"content\":{\"connectorIds\":[],\"side\":\"BOTTOM\"},\"type\":\"ConnectorPlacement.EquallySpacedRectSide\",\"uuid\":\"6f2036ec-938c-44a9-afb7-06059bf5c36d\"},{\"content\":{\"connectorIds\":[\"In1\"],\"side\":\"HIDDEN\"},\"type\":\"ConnectorPlacement.EquallySpacedRectSide\",\"uuid\":\"75439cfd-37c7-42f5-ab17-1be2c2229a41\"}]},\"type\":\"ConnectorPlacement.EquallySpacedConnector\",\"uuid\":\"b6b0d473-12c9-4a38-8dee-bffc8352e44f\"}],\"packageUris\":[\"http://schema.mathworks.com/mf0/Connector/R2020b\"],\"version\":\"1.0\"}"
  UIF_LED_ColorCode : ModelReference  ModelNameDialog=UIF_LED_ColorCode  SimulationMode=Normal  ScheduleRates=on  ModelEventPortInfo=P:D1[-2][0][0]  ModelReferenceVersion=1.5
      settings: PortSchema="{\"entries\":[{\"content\":{\"headerSize\":38,\"margin\":15,\"minimumSpacing\":25,\"sides\":[{\"content\":{\"connectorIds\":[\"In1\",\"In2\"]},\"type\":\"ConnectorPlacement.EquallySpacedRectSide\",\"uuid\":\"9fafbac4-d9ff-4bef-9686-25ce946f922a\"},{\"content\":{\"connectorIds\":[],\"side\":\"RIGHT\"},\"type\":\"ConnectorPlacement.EquallySpacedRectSide\",\"uuid\":\"64958763-52cc-4c3d-9da1-de7e7fca94ff\"},{\"content\":{\"connectorIds\":[],\"side\":\"TOP\"},\"type\":\"ConnectorPlacement.EquallySpacedRectSide\",\"uuid\":\"29c78429-a934-4b6b-906c-5a3963e1854a\"},{\"content\":{\"connectorIds\":[\"In3\"],\"side\":\"HIDDEN\"},\"type\":\"ConnectorPlacement.EquallySpacedRectSide\",\"uuid\":\"d382be67-5be4-4eda-9276-c603c8248b01\"}]},\"type\":\"ConnectorPlacement.EquallySpacedConnector\",\"uuid\":\"b6b0d473-12c9-4a38-8dee-bffc8352e44f\"}],\"packageUris\":[\"http://schema.mathworks.com/mf0/Connector/R2020b\"],\"version\":\"1.0\"}"
  Bus Element Out1 : Outport  PortName=SW1_Read
  Bus Element Out2 : Outport  Port=2  PortName=SW2_Read
  wires:
  Bus Element In1/1 -> UIF_LED_ColorCode/1
  Bus Element In2/1 -> UIF_LED_ColorCode/2
  UIF_BUT_Read/1 -> Bus Element Out1/1
  UIF_BUT_Read/2 -> Bus Element Out2/1
